simulink model "lqr_period_ideal_simu"  (R2015a)
settings: Solver=ode45  SolverMode=SingleTasking  StartTime=0.0  StopTime=simu.time  RelTol=1e-3
values from neighbouring files (symbols this model uses):
  ctrl_K = K    [lqr_period_ideal_m.m]
  ctrl_N = N_bar    [lqr_period_ideal_m.m]
  g_Ts = i    [lqr_period_ideal_m.m]    (also in lqr_period_with_abitary_reference.m = 100)
  ref_mag = 1.0    (= 1)    [lqr_period_ideal_m.m]
undefined symbols (not defined in the file or in its folder): simu
settings Model: CovSFcnEnable=off  ExtModeTrigMode=oneshot  ExtModeArmWhenConnect=off  Creator=The MathWorks Inc.  LastModifiedBy=Xiaotian
settings DataIOCC: LimitDataPoints=off  SaveOutput=off  SignalLogging=off  DSMLogging=off  SaveTime=off  SignalLoggingName=sigsOut
settings OptimizationCC: BooleanDataType=off  ExpressionDepthLimit=2147483647  InitFltsAndDblsToZero=on
settings DebuggingCC: SaveWithParameterizedLinksMsg=none  UnderspecifiedInitializationDetection=Classic  MergeDetectMultiDrivingBlocksExec=none  SignalResolutionControl=TryResolveAllWithWarning  MultiTaskDSMMsg=warning  MultiTaskCondExecSysMsg=none  IntegerOverflowMsg=none  FcnCallInpInsideContextMsg=UseLocalSettings  StateNameClashWarn=warning  IntegerSaturationMsg=none
settings HardwareCC: TargetUnknown=on
settings GRTTargetCC: TargetFcnLib=ansi_tfl_tmw.mat  CombineOutputUpdateFcns=off  GRTInterface=on

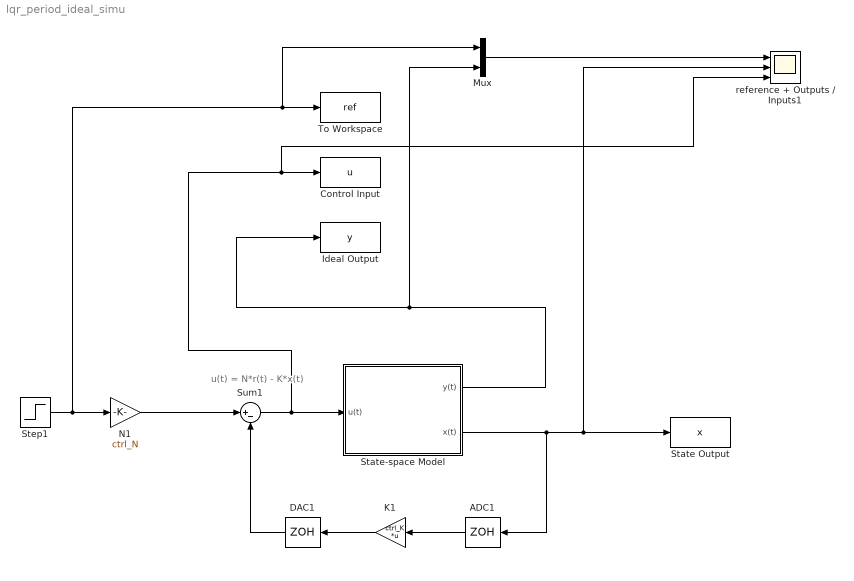
== system lqr_period_ideal_simu ==
  note: u(t) = N*r(t) - K*x(t)
  ADC1 : ZeroOrderHold  SampleTime=g_Ts
  Control Input : ToWorkspace  VariableName=u  SampleTime=simu.samlping_time
      settings: MaxDataPoints=Inf
  DAC1 : ZeroOrderHold  SampleTime=g_Ts
  Ideal Output : ToWorkspace  VariableName=y  SampleTime=simu.samlping_time
      settings: MaxDataPoints=Inf
  K1 : Gain  Gain=ctrl_K  Multiplication=Matrix(K*u)
  Mux : Mux  Inputs=2
  N1 : Gain  Gain=ctrl_N
  State Output : ToWorkspace  VariableName=x  SampleTime=simu.samlping_time
      settings: MaxDataPoints=Inf
  State-space Model : Subsystem  mask(State-space){A=0, B=0, C=0, D=0}
      mask help:
      | A state-space block using raw Simulink elements.
      | Internal states are exposed to use.
  Step1 : Step  Time=0  After=ref_mag  SampleTime=0
  Sum1 : Sum  Inputs=|+-
  To Workspace : ToWorkspace  VariableName=ref  SampleTime=simu.samlping_time
  reference + Outputs / Inputs1 : Scope  NumInputPorts=3
      settings: TimeRange=1  YMin=-0.25~-600~-5  YMax=3~200~5  DataFormat=Structure  SampleInput=on  SampleTime=simu.samlping_time
  wires:
  State-space Model/1(y(t)) -> Mux/2, Ideal Output/1
  State-space Model/2(x(t)) -> State Output/1, reference + Outputs / Inputs1/2, ADC1/1
  ADC1/1 -> K1/1
  K1/1 -> DAC1/1
  DAC1/1 -> Sum1/2
  Sum1/1 -> reference + Outputs / Inputs1/3, Control Input/1, State-space Model/1(u(t))
  N1/1 -> Sum1/1
  Step1/1 -> Mux/1, To Workspace/1, N1/1
  Mux/1 -> reference + Outputs / Inputs1/1

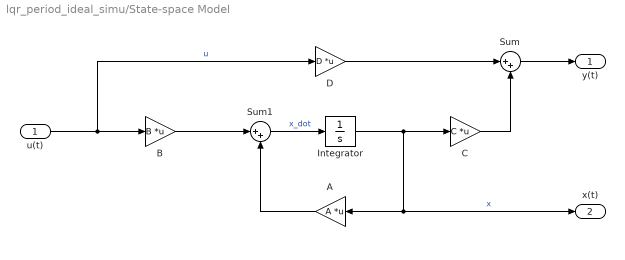
== system lqr_period_ideal_simu/State-space Model ==
  u(t) : Inport
  A : Gain  Gain=A  Multiplication=Matrix(K*u)
  B : Gain  Gain=B  Multiplication=Matrix(K*u)
  C : Gain  Gain=C  Multiplication=Matrix(K*u)
  D : Gain  Gain=D  Multiplication=Matrix(K*u)
  Integrator : Integrator
  Sum : Sum  Inputs=|++
  Sum1 : Sum  Inputs=|++
  y(t) : Outport
  x(t) : Outport  Port=2
  wires:
  u(t)/1 -> D/1, B/1  "u"
  B/1 -> Sum1/1
  A/1 -> Sum1/2
  Sum1/1 -> Integrator/1  "x_dot"
  Integrator/1 -> A/1, x(t)/1, C/1  "x"
  D/1 -> Sum/1
  C/1 -> Sum/2
  Sum/1 -> y(t)/1
